simulink model "test_pfb_real"  (Simulink 6.2)
settings: Solver=ode45  StartTime=0.0  StopTime=10.0  RelTol=1e-3
libraries: xbsIndex_r3 x123, casper_library x8
(part 2 of 2)

== system test_pfb_real/pfb_fir_real/pol1_in2_last_tap/pfb_real_add_tree ==
  din : Inport  Port=1  LatchInput=off
  sync : Inport  Port=2  LatchInput=off
  Reint0 : xbsIndex_r3/Reinterpret  force_arith_type=on  arith_type="Signed  (2's comp)"  force_bin_pt=on  bin_pt=CoeffBitWidth + BitWidthIn - 2  force_valid=on
  Reint1 : xbsIndex_r3/Reinterpret  force_arith_type=on  arith_type="Signed  (2's comp)"  force_bin_pt=on  bin_pt=CoeffBitWidth + BitWidthIn - 2  force_valid=on
  Slice0 : xbsIndex_r3/Slice  mode=Upper Bit Location + Width  nbits=CoeffBitWidth + BitWidthIn  bit1=-0*(CoeffBitWidth + BitWidthIn)  base1=MSB of Input  bit0=0  base0=MSB of Input  boolean_output=off  explicit_period=off  period=1  dbl_ovrd=off
  Slice1 : xbsIndex_r3/Slice  mode=Upper Bit Location + Width  nbits=CoeffBitWidth + BitWidthIn  bit1=-1*(CoeffBitWidth + BitWidthIn)  base1=MSB of Input  bit0=0  base0=MSB of Input  boolean_output=off  explicit_period=off  period=1  dbl_ovrd=off
  adder_tree1 : Subsystem  AncestorBlock=casper_library/Misc/adder_tree  mask(adder_tree){n_inputs=2, latency=1}
      mask prompts: n_inputs "Number of Inputs"; latency "Add Latency"
      mask help: Sums all inputs using a tree of adds and delays.
      mask init:
      | adder_tree_init(gcb, ...
      |     'n_inputs', n_inputs, ...
      |     'latency', latency);
      settings: AttributesFormatString=latency 1
      mask Help: eval('xlWeb([getenv(''MLIB_ROOT''), ''\doc\html\sp_adder_tree\sp_adder_tree.html''])')
  convert1 : xbsIndex_r3/Convert  arith_type="Signed  (2's comp)"  n_bits=BitWidthOut  bin_pt=BitWidthOut-1  quantization=Truncate  overflow=Saturate  latency=add_latency  explicit_period=off  period=1  dbl_ovrd=off  show_param=off  inserted_by_tool=off  pipeline=off
      settings: xl_area=[0, 0, 0, 0, 0, 0, 0]
  delay1 : xbsIndex_r3/Delay  latency=1  reg_retiming=off  explicit_period=off  period=1  en=off  accept_only_valid=off  init_zero=on  dbl_ovrd=off  show_param=off
      settings: xl_area=[0, 0, 0, 0, 0, 0, 0]
  scale1 : xbsIndex_r3/Scale  scale_factor=-2  explicit_period=off  period=1  dbl_ovrd=off
  dout : Outport
  sync_out : Outport  Port=2
  wires:
  adder_tree1/2(dout) -> scale1/1
  scale1/1 -> convert1/1
  convert1/1 -> dout/1
  sync/1 -> adder_tree1/1(sync)
  adder_tree1/1(sync_out) -> delay1/1
  delay1/1 -> sync_out/1
  din/1 -> Slice0/1, Slice1/1
  Slice0/1 -> Reint0/1
  Reint0/1 -> adder_tree1/2(din1)
  Slice1/1 -> Reint1/1
  Reint1/1 -> adder_tree1/3(din2)

== system test_pfb_real/pfb_fir_real/pol1_in3_first_tap/delay ==
  In1 : Inport  Port=1  LatchInput=off
  delay_bram : casper_library/Delays/delay_bram  DelayLen=2^(PFBSize-n_inputs)  bram_latency=bram_latency
  Out1 : Outport
  wires:
  In1/1 -> delay_bram/1
  delay_bram/1 -> Out1/1

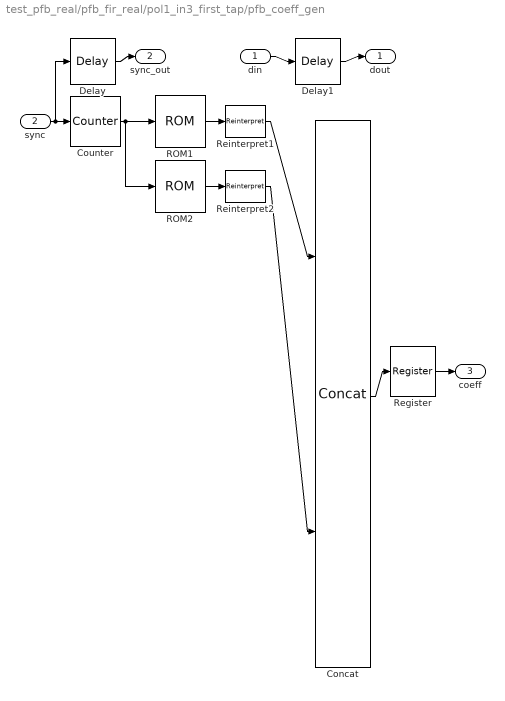
== system test_pfb_real/pfb_fir_real/pol1_in3_first_tap/pfb_coeff_gen ==
  din : Inport  Port=1  LatchInput=off
  sync : Inport  Port=2  LatchInput=off
  Concat : xbsIndex_r3/Concat  num_inputs=2  explicit_period=off  period=1  dbl_ovrd=off
  Counter : xbsIndex_r3/Counter  cnt_type=Free Running  n_bits=6  bin_pt=0  arith_type=Unsigned  start_count=0  cnt_to=Inf  cnt_by_val=1  operation=Up  explicit_period=on  period=1  load_pin=off  rst=on  en=off  dbl_ovrd=off  show_param=off  use_rpm=on  gen_core=off
      settings: xl_area=[0, 0, 0, 0, 0, 0, 0]
  Delay : xbsIndex_r3/Delay  latency=bram_latency+1  reg_retiming=off  explicit_period=off  period=1  en=off  accept_only_valid=off  init_zero=on  dbl_ovrd=off  show_param=off
      settings: xl_area=[0, 0, 0, 0, 0, 0, 0]
  Delay1 : xbsIndex_r3/Delay  latency=3  reg_retiming=off  explicit_period=off  period=1  en=off  accept_only_valid=off  init_zero=on  dbl_ovrd=off  show_param=off
      settings: xl_area=[0, 0, 0, 0, 0, 0, 0]
  ROM1 : xbsIndex_r3/ROM  depth=64  initVector=[0.000630953074967074 0.00194826894833786 0.00338469890746931 0.00499674871201254 0.00684307086604839 0.00898400011986041 0.0114810647329688 0.0143964771252502 0.0177926077539941 0.0217314462363914 0.0262740538874815 0.0314800119615337 0.0374068699689719 0.0441095984903377 0.0516400509227496 0.0600464385724883 0.0693728234496303 0.0796586330272857 0.0909382010994727 0.103240338708793 0.116587938918932 0.130997618978996 0.146479403168405 0.163036449324448 0.180664821741746 0.199353312796187 0.219083315287929 0.239828747121581 0.26155602954962 0.284224119800518 0.307784598499137 0.332181811866997 0.357353068267332 0.383228888237845 0.409733306736097 0.436784225911947 0.464293816321626 0.492168964112259 0.520311761336936 0.548620036211956 0.576987919802344 0.605306445322013 0.633464175963314 0.661347856929703 0.688843087136625 0.715835005871452 0.742208989564828 0.767851353724256 0.79265005501725 0.816495388466347 0.839280674732153 0.860902932513311 0.881263531183556 0.900268818915202 0.917830721704562 0.933867308916738 0.94830332120334 0.961070656915272 0.972108813431647 0.981365280152876 0.988795880258447 0.994365058705201 0.99804611433694 0.99982137438808]  arith_type="Signed  (2's comp)"  n_bits=8  bin_pt=7  latency=2  init_zero=on  explicit_period=off  period=1  rst=off  init_reg=0  en=off  dbl_ovrd=off  show_param=on  distributed_mem=on  use_rpm=on  gen_core=off
      settings: xl_area=[0, 0, 0, 0, 0, 0, 0]
  ROM2 : xbsIndex_r3/ROM  depth=64  initVector=[0.999682310089356 0.997629592519081 0.993673088285716 0.987831795072995 0.980133717524106 0.970615684382962 0.95932310824487 0.946309689692593 0.931637068003491 0.915374421005982 0.897598017035832 0.878390722291939 0.857841467214529 0.836044675803548 0.813099662059281 0.789109997958721 0.764182857578294 0.738428342134668 0.711958790839383 0.684888082548983 0.65733093323971 0.629402194344284 0.601216156957919 0.572885866851882 0.544522455126173 0.516234489189376 0.488127348574552 0.460302629886806 0.43285758493267 0.405884595805773 0.379470690399712 0.353697101490091 0.328638872176137 0.304364510100978 0.2809356924816 0.258407023577912 0.236825845818455 0.216232105381412 0.196658272607163 0.17812931719593 0.16066273772465 0.144268644604162 0.128949895194702 0.114702279407366 0.101514753745028 0.0893697213808225 0.0782433555386214 0.0681059631304454 0.0589223853227576 0.0506524314492739 0.0432513424640886 0.0366702799371903 0.0308568364361624 0.0257555630140703 0.0213085094349984 0.0174557727158867 0.0141360495464024 0.0112871881674359 0.00884673534303718 0.00675247414947995 0.00494294842769327 0.0033579699002687 0.00193910414012047 0.000630131792892409]  arith_type="Signed  (2's comp)"  n_bits=8  bin_pt=7  latency=2  init_zero=on  explicit_period=off  period=1  rst=off  init_reg=0  en=off  dbl_ovrd=off  show_param=on  distributed_mem=on  use_rpm=on  gen_core=off
      settings: xl_area=[0, 0, 0, 0, 0, 0, 0]
  Register : xbsIndex_r3/Register  init=0  reg_only_valid=off  explicit_period=off  period=1  rst=off  en=off  out_en=off  dbl_ovrd=off  show_param=off
      settings: xl_area=[0, 0, 0, 0, 0, 0, 0]
  Reinterpret1 : xbsIndex_r3/Reinterpret  force_arith_type=on  arith_type=Unsigned  force_bin_pt=on  bin_pt=0  force_valid=on
  Reinterpret2 : xbsIndex_r3/Reinterpret  force_arith_type=on  arith_type=Unsigned  force_bin_pt=on  bin_pt=0  force_valid=on
  dout : Outport
  sync_out : Outport  Port=2
  coeff : Outport  Port=3
  wires:
  din/1 -> Delay1/1
  Delay1/1 -> dout/1
  sync/1 -> Counter/1, Delay/1
  Delay/1 -> sync_out/1
  Concat/1 -> Register/1
  Register/1 -> coeff/1
  Counter/1 -> ROM1/1, ROM2/1
  ROM1/1 -> Reinterpret1/1
  Reinterpret1/1 -> Concat/1
  ROM2/1 -> Reinterpret2/1
  Reinterpret2/1 -> Concat/2

== system test_pfb_real/pfb_fir_real/pol1_in3_last_tap/pfb_real_add_tree ==
  din : Inport  Port=1  LatchInput=off
  sync : Inport  Port=2  LatchInput=off
  Reint0 : xbsIndex_r3/Reinterpret  force_arith_type=on  arith_type="Signed  (2's comp)"  force_bin_pt=on  bin_pt=CoeffBitWidth + BitWidthIn - 2  force_valid=on
  Reint1 : xbsIndex_r3/Reinterpret  force_arith_type=on  arith_type="Signed  (2's comp)"  force_bin_pt=on  bin_pt=CoeffBitWidth + BitWidthIn - 2  force_valid=on
  Slice0 : xbsIndex_r3/Slice  mode=Upper Bit Location + Width  nbits=CoeffBitWidth + BitWidthIn  bit1=-0*(CoeffBitWidth + BitWidthIn)  base1=MSB of Input  bit0=0  base0=MSB of Input  boolean_output=off  explicit_period=off  period=1  dbl_ovrd=off
  Slice1 : xbsIndex_r3/Slice  mode=Upper Bit Location + Width  nbits=CoeffBitWidth + BitWidthIn  bit1=-1*(CoeffBitWidth + BitWidthIn)  base1=MSB of Input  bit0=0  base0=MSB of Input  boolean_output=off  explicit_period=off  period=1  dbl_ovrd=off
  adder_tree1 : Subsystem  AncestorBlock=casper_library/Misc/adder_tree  mask(adder_tree){n_inputs=2, latency=1}
      mask prompts: n_inputs "Number of Inputs"; latency "Add Latency"
      mask help: Sums all inputs using a tree of adds and delays.
      mask init:
      | adder_tree_init(gcb, ...
      |     'n_inputs', n_inputs, ...
      |     'latency', latency);
      settings: AttributesFormatString=latency 1
      mask Help: eval('xlWeb([getenv(''MLIB_ROOT''), ''\doc\html\sp_adder_tree\sp_adder_tree.html''])')
  convert1 : xbsIndex_r3/Convert  arith_type="Signed  (2's comp)"  n_bits=BitWidthOut  bin_pt=BitWidthOut-1  quantization=Truncate  overflow=Saturate  latency=add_latency  explicit_period=off  period=1  dbl_ovrd=off  show_param=off  inserted_by_tool=off  pipeline=off
      settings: xl_area=[0, 0, 0, 0, 0, 0, 0]
  delay1 : xbsIndex_r3/Delay  latency=1  reg_retiming=off  explicit_period=off  period=1  en=off  accept_only_valid=off  init_zero=on  dbl_ovrd=off  show_param=off
      settings: xl_area=[0, 0, 0, 0, 0, 0, 0]
  scale1 : xbsIndex_r3/Scale  scale_factor=-2  explicit_period=off  period=1  dbl_ovrd=off
  dout : Outport
  sync_out : Outport  Port=2
  wires:
  adder_tree1/2(dout) -> scale1/1
  scale1/1 -> convert1/1
  convert1/1 -> dout/1
  sync/1 -> adder_tree1/1(sync)
  adder_tree1/1(sync_out) -> delay1/1
  delay1/1 -> sync_out/1
  din/1 -> Slice0/1, Slice1/1
  Slice0/1 -> Reint0/1
  Reint0/1 -> adder_tree1/2(din1)
  Slice1/1 -> Reint1/1
  Reint1/1 -> adder_tree1/3(din2)

== system test_pfb_real/pfb_fir_real/pol1_in4_first_tap/delay ==
  In1 : Inport  Port=1  LatchInput=off
  delay_bram : casper_library/Delays/delay_bram  DelayLen=2^(PFBSize-n_inputs)  bram_latency=bram_latency
  Out1 : Outport
  wires:
  In1/1 -> delay_bram/1
  delay_bram/1 -> Out1/1

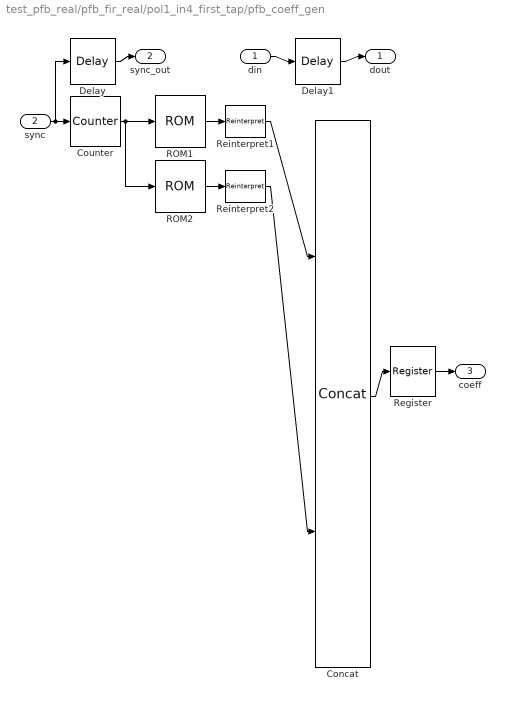
== system test_pfb_real/pfb_fir_real/pol1_in4_first_tap/pfb_coeff_gen ==
  din : Inport  Port=1  LatchInput=off
  sync : Inport  Port=2  LatchInput=off
  Concat : xbsIndex_r3/Concat  num_inputs=2  explicit_period=off  period=1  dbl_ovrd=off
  Counter : xbsIndex_r3/Counter  cnt_type=Free Running  n_bits=6  bin_pt=0  arith_type=Unsigned  start_count=0  cnt_to=Inf  cnt_by_val=1  operation=Up  explicit_period=on  period=1  load_pin=off  rst=on  en=off  dbl_ovrd=off  show_param=off  use_rpm=on  gen_core=off
      settings: xl_area=[0, 0, 0, 0, 0, 0, 0]
  Delay : xbsIndex_r3/Delay  latency=bram_latency+1  reg_retiming=off  explicit_period=off  period=1  en=off  accept_only_valid=off  init_zero=on  dbl_ovrd=off  show_param=off
      settings: xl_area=[0, 0, 0, 0, 0, 0, 0]
  Delay1 : xbsIndex_r3/Delay  latency=3  reg_retiming=off  explicit_period=off  period=1  en=off  accept_only_valid=off  init_zero=on  dbl_ovrd=off  show_param=off
      settings: xl_area=[0, 0, 0, 0, 0, 0, 0]
  ROM1 : xbsIndex_r3/ROM  depth=64  initVector=[0.000952112049876172 0.00229404313369537 0.00376898909202097 0.00543403446197535 0.00734829686255785 0.00957245610930944 0.0121682599756256 0.0151980102829498 0.0187240332059367 0.02280813785269 0.0275110673226984 0.0328919465546884 0.0390077313521386 0.0459126630147819 0.0536577330094605 0.0622901620828955 0.0718528981522823 0.082384137207404 0.0939168713207625 0.106478467690925 0.120090282440038 0.134767312650712 0.150517889861922 0.167343417950188 0.185238158003244 0.204189062451155 0.224175660356992 0.245169995388492 0.267136617596671 0.29003262972014 0.313807788318118 0.33840465961421 0.363758829510161 0.389799166807495 0.416448138258519 0.443622173660013 0.471232078806306 0.499183493736657 0.52737739334791 0.555710627100403 0.584076494225782 0.612365350552457 0.64046524280024 0.668262565962614 0.695642739194903 0.72249089546113 0.748692580063041 0.774134453082666 0.79870499071584 0.822295180458815 0.844799205133662 0.866115110800595 0.886145453706144 0.904797921554624 0.921985924565623 0.937629151990793 0.951654090007714 0.963994497184924 0.974591834018397 0.983395643373337 0.99036387902361 0.995463179861633 0.998669087751084 0.99996620741033]  arith_type="Signed  (2's comp)"  n_bits=8  bin_pt=7  latency=2  init_zero=on  explicit_period=off  period=1  rst=off  init_reg=0  en=off  dbl_ovrd=off  show_param=on  distributed_mem=on  use_rpm=on  gen_core=off
      settings: xl_area=[0, 0, 0, 0, 0, 0, 0]
  ROM2 : xbsIndex_r3/ROM  depth=64  initVector=[0.999348307142622 0.996818359666656 0.992388522744416 0.986080059749065 0.977923200760209 0.967956945213987 0.95622880756732 0.94279450785618 0.927717609433444 0.911069106559645 0.892926964886701 0.873375618217632 0.852505425241652 0.830412090231434 0.807196051945602 0.782961845202524 0.75781743977972 0.731873561445143 0.705243000041136 0.678039909618233 0.650379105653632 0.622375364387898 0.594142729273431 0.565793829449825 0.537439215045239 0.509186713950316 0.481140814523328 0.453402078463767 0.426066587838342 0.39922542996049 0.372964223514345 0.347362688979257 0.322494266054191 0.298425780405488 0.275217161669781 0.25292121423935 0.231583441943243 0.211241927317438 0.191927265734484 0.173662554240905 0.156463434532477 0.140338189086687 0.125287889071402 0.111306592262291 0.0983815888317304 0.0864936925217694 0.0756175743858404 0.065722135980832 0.0567709186151387 0.0487225450114299 0.041531189526942 0.0351470728906169 0.0295169772666643 0.0245847773390881 0.0202919830320737 0.0165782894372938 0.0133821295112371 0.0106412251334151 0.00829313217926387 0.00627577535895479 0.00452796870411217 0.00298991774727936 0.0016036996323074 0.000313717615839077]  arith_type="Signed  (2's comp)"  n_bits=8  bin_pt=7  latency=2  init_zero=on  explicit_period=off  period=1  rst=off  init_reg=0  en=off  dbl_ovrd=off  show_param=on  distributed_mem=on  use_rpm=on  gen_core=off
      settings: xl_area=[0, 0, 0, 0, 0, 0, 0]
  Register : xbsIndex_r3/Register  init=0  reg_only_valid=off  explicit_period=off  period=1  rst=off  en=off  out_en=off  dbl_ovrd=off  show_param=off
      settings: xl_area=[0, 0, 0, 0, 0, 0, 0]
  Reinterpret1 : xbsIndex_r3/Reinterpret  force_arith_type=on  arith_type=Unsigned  force_bin_pt=on  bin_pt=0  force_valid=on
  Reinterpret2 : xbsIndex_r3/Reinterpret  force_arith_type=on  arith_type=Unsigned  force_bin_pt=on  bin_pt=0  force_valid=on
  dout : Outport
  sync_out : Outport  Port=2
  coeff : Outport  Port=3
  wires:
  din/1 -> Delay1/1
  Delay1/1 -> dout/1
  sync/1 -> Counter/1, Delay/1
  Delay/1 -> sync_out/1
  Concat/1 -> Register/1
  Register/1 -> coeff/1
  Counter/1 -> ROM1/1, ROM2/1
  ROM1/1 -> Reinterpret1/1
  Reinterpret1/1 -> Concat/1
  ROM2/1 -> Reinterpret2/1
  Reinterpret2/1 -> Concat/2

== system test_pfb_real/pfb_fir_real/pol1_in4_last_tap/pfb_real_add_tree ==
  din : Inport  Port=1  LatchInput=off
  sync : Inport  Port=2  LatchInput=off
  Reint0 : xbsIndex_r3/Reinterpret  force_arith_type=on  arith_type="Signed  (2's comp)"  force_bin_pt=on  bin_pt=CoeffBitWidth + BitWidthIn - 2  force_valid=on
  Reint1 : xbsIndex_r3/Reinterpret  force_arith_type=on  arith_type="Signed  (2's comp)"  force_bin_pt=on  bin_pt=CoeffBitWidth + BitWidthIn - 2  force_valid=on
  Slice0 : xbsIndex_r3/Slice  mode=Upper Bit Location + Width  nbits=CoeffBitWidth + BitWidthIn  bit1=-0*(CoeffBitWidth + BitWidthIn)  base1=MSB of Input  bit0=0  base0=MSB of Input  boolean_output=off  explicit_period=off  period=1  dbl_ovrd=off
  Slice1 : xbsIndex_r3/Slice  mode=Upper Bit Location + Width  nbits=CoeffBitWidth + BitWidthIn  bit1=-1*(CoeffBitWidth + BitWidthIn)  base1=MSB of Input  bit0=0  base0=MSB of Input  boolean_output=off  explicit_period=off  period=1  dbl_ovrd=off
  adder_tree1 : Subsystem  AncestorBlock=casper_library/Misc/adder_tree  mask(adder_tree){n_inputs=2, latency=1}
      mask prompts: n_inputs "Number of Inputs"; latency "Add Latency"
      mask help: Sums all inputs using a tree of adds and delays.
      mask init:
      | adder_tree_init(gcb, ...
      |     'n_inputs', n_inputs, ...
      |     'latency', latency);
      settings: AttributesFormatString=latency 1
      mask Help: eval('xlWeb([getenv(''MLIB_ROOT''), ''\doc\html\sp_adder_tree\sp_adder_tree.html''])')
  convert1 : xbsIndex_r3/Convert  arith_type="Signed  (2's comp)"  n_bits=BitWidthOut  bin_pt=BitWidthOut-1  quantization=Truncate  overflow=Saturate  latency=add_latency  explicit_period=off  period=1  dbl_ovrd=off  show_param=off  inserted_by_tool=off  pipeline=off
      settings: xl_area=[0, 0, 0, 0, 0, 0, 0]
  delay1 : xbsIndex_r3/Delay  latency=1  reg_retiming=off  explicit_period=off  period=1  en=off  accept_only_valid=off  init_zero=on  dbl_ovrd=off  show_param=off
      settings: xl_area=[0, 0, 0, 0, 0, 0, 0]
  scale1 : xbsIndex_r3/Scale  scale_factor=-2  explicit_period=off  period=1  dbl_ovrd=off
  dout : Outport
  sync_out : Outport  Port=2
  wires:
  adder_tree1/2(dout) -> scale1/1
  scale1/1 -> convert1/1
  convert1/1 -> dout/1
  sync/1 -> adder_tree1/1(sync)
  adder_tree1/1(sync_out) -> delay1/1
  delay1/1 -> sync_out/1
  din/1 -> Slice0/1, Slice1/1
  Slice0/1 -> Reint0/1
  Reint0/1 -> adder_tree1/2(din1)
  Slice1/1 -> Reint1/1
  Reint1/1 -> adder_tree1/3(din2)

== system test_pfb_real/pfb_fir_real/pol1_in1_last_tap/pfb_real_add_tree/adder_tree1 ==
  sync : Inport  Port=1  LatchInput=off
  din1 : Inport  Port=2  LatchInput=off
  din2 : Inport  Port=3  LatchInput=off
  addr1 : xbsIndex_r3/AddSub  mode=Addition  precision=Full  arith_type=Unsigned  n_bits=8  bin_pt=2  quantization=Truncate  overflow=Wrap  latency=1  explicit_period=off  period=1  use_carryin=off  use_carryout=off  en=off  dbl_ovrd=off  show_param=off  use_core=on  pipeline=on  use_rpm=on  gen_core=off
      settings: xl_area=[0, 0, 0, 0, 0, 0, 0]
  sync_delay : xbsIndex_r3/Delay  latency=1  reg_retiming=off  explicit_period=off  period=1  en=off  accept_only_valid=off  init_zero=on  dbl_ovrd=off  show_param=off
      settings: xl_area=[0, 0, 0, 0, 0, 0, 0]
  sync_out : Outport
  dout : Outport  Port=2
  wires:
  sync/1 -> sync_delay/1
  sync_delay/1 -> sync_out/1
  din1/1 -> addr1/1
  din2/1 -> addr1/2
  addr1/1 -> dout/1

== system test_pfb_real/pfb_fir_real/pol1_in2_last_tap/pfb_real_add_tree/adder_tree1 ==
  sync : Inport  Port=1  LatchInput=off
  din1 : Inport  Port=2  LatchInput=off
  din2 : Inport  Port=3  LatchInput=off
  addr1 : xbsIndex_r3/AddSub  mode=Addition  precision=Full  arith_type=Unsigned  n_bits=8  bin_pt=2  quantization=Truncate  overflow=Wrap  latency=1  explicit_period=off  period=1  use_carryin=off  use_carryout=off  en=off  dbl_ovrd=off  show_param=off  use_core=on  pipeline=on  use_rpm=on  gen_core=off
      settings: xl_area=[0, 0, 0, 0, 0, 0, 0]
  sync_delay : xbsIndex_r3/Delay  latency=1  reg_retiming=off  explicit_period=off  period=1  en=off  accept_only_valid=off  init_zero=on  dbl_ovrd=off  show_param=off
      settings: xl_area=[0, 0, 0, 0, 0, 0, 0]
  sync_out : Outport
  dout : Outport  Port=2
  wires:
  sync/1 -> sync_delay/1
  sync_delay/1 -> sync_out/1
  din1/1 -> addr1/1
  din2/1 -> addr1/2
  addr1/1 -> dout/1

== system test_pfb_real/pfb_fir_real/pol1_in3_last_tap/pfb_real_add_tree/adder_tree1 ==
  sync : Inport  Port=1  LatchInput=off
  din1 : Inport  Port=2  LatchInput=off
  din2 : Inport  Port=3  LatchInput=off
  addr1 : xbsIndex_r3/AddSub  mode=Addition  precision=Full  arith_type=Unsigned  n_bits=8  bin_pt=2  quantization=Truncate  overflow=Wrap  latency=1  explicit_period=off  period=1  use_carryin=off  use_carryout=off  en=off  dbl_ovrd=off  show_param=off  use_core=on  pipeline=on  use_rpm=on  gen_core=off
      settings: xl_area=[0, 0, 0, 0, 0, 0, 0]
  sync_delay : xbsIndex_r3/Delay  latency=1  reg_retiming=off  explicit_period=off  period=1  en=off  accept_only_valid=off  init_zero=on  dbl_ovrd=off  show_param=off
      settings: xl_area=[0, 0, 0, 0, 0, 0, 0]
  sync_out : Outport
  dout : Outport  Port=2
  wires:
  sync/1 -> sync_delay/1
  sync_delay/1 -> sync_out/1
  din1/1 -> addr1/1
  din2/1 -> addr1/2
  addr1/1 -> dout/1

== system test_pfb_real/pfb_fir_real/pol1_in4_last_tap/pfb_real_add_tree/adder_tree1 ==
  sync : Inport  Port=1  LatchInput=off
  din1 : Inport  Port=2  LatchInput=off
  din2 : Inport  Port=3  LatchInput=off
  addr1 : xbsIndex_r3/AddSub  mode=Addition  precision=Full  arith_type=Unsigned  n_bits=8  bin_pt=2  quantization=Truncate  overflow=Wrap  latency=1  explicit_period=off  period=1  use_carryin=off  use_carryout=off  en=off  dbl_ovrd=off  show_param=off  use_core=on  pipeline=on  use_rpm=on  gen_core=off
      settings: xl_area=[0, 0, 0, 0, 0, 0, 0]
  sync_delay : xbsIndex_r3/Delay  latency=1  reg_retiming=off  explicit_period=off  period=1  en=off  accept_only_valid=off  init_zero=on  dbl_ovrd=off  show_param=off
      settings: xl_area=[0, 0, 0, 0, 0, 0, 0]
  sync_out : Outport
  dout : Outport  Port=2
  wires:
  sync/1 -> sync_delay/1
  sync_delay/1 -> sync_out/1
  din1/1 -> addr1/1
  din2/1 -> addr1/2
  addr1/1 -> dout/1
